simulink model "VCU_TDN"  (R2020a)
settings: Solver=FixedStepDiscrete  StartTime=0.0  StopTime=10.0  FixedStep=0.001  RelTol=1e-3  EnableMultiTasking=on
InitFcn:
  | EcoCoder_PreCheckLic();
undefined symbols (not defined in the file or in its folder): h, km
libraries: CoderSF_BSW_Libs x139, simulink x1, SF_CanService_Libs x1
(part 1 of 2)
settings Model: Creator=timot  LastModifiedBy=timot
settings DataIOCC: SaveFormat=Structure  SignalLoggingSaveFormat=ModelDataLogs  SaveOutput=off  SignalLogging=off  DSMLogging=off  SaveTime=off  ReturnWorkspaceOutputs=off
settings OptimizationCC: DefaultParameterBehavior=Inlined  InlineInvariantSignals=on  EnhancedBackFolding=on  StrengthReduction=on  EnableMemcpy=off  PassReuseOutputArgsAs=Individual arguments  EfficientFloat2IntCast=on  LifeSpan=1  SimCompilerOptimization=on  OptimizeBlockOrder=speed  DifferentSizesBufferReuse=on  EfficientTunableParamExpr=on
settings DebuggingCC: AlgebraicLoopMsg=none  ArtificialAlgebraicLoopMsg=none  SaveWithDisabledLinksMsg=none  SaveWithParameterizedLinksMsg=none  CheckSSInitialOutputMsg=off  UnderspecifiedInitializationDetection=Classic  SignalResolutionControl=TryResolveAll  BlockPriorityViolationMsg=error  MinStepSizeMsg=none  InheritedTsInSrcMsg=none  MultiTaskDSMMsg=none  MultiTaskCondExecSysMsg=none  MultiTaskRateTransMsg=warning  TasksWithSamePriorityMsg=none  SigSpecEnsureSampleTimeMsg=none  IntegerOverflowMsg=error  Int32ToFloatConvMsg=none  ParameterPrecisionLossMsg=none  ParameterTunabilityLossMsg=none  FixptConstOverflowMsg=error  FcnCallInpInsideContextMsg=warning  UnconnectedInputMsg=error  UnconnectedOutputMsg=error  UnconnectedLineMsg=error  FrameProcessingCompatibilityMsg=none  BusObjectLabelMismatch=none  RootOutportRequireBusObject=none  UnknownTsInhSupMsg=none  ModelReferenceDataLoggingMessage=none  OperatingPointInterfaceChecksumMismatchMsg=none  SFUnusedDataAndEventsDiag=none  SFUnexpectedBacktrackingDiag=none  SFInvalidInputDataAccessInChartInitDiag=none  SFNoUnconditionalDefaultTransitionDiag=none  SFTransitionOutsideNaturalParentDiag=none  SFUnreachableExecutionPathDiag=none  SFMachineParentedDataDiag=error
settings HardwareCC: ProdBitPerPointer=32  ProdBitPerSizeT=32  ProdBitPerPtrDiffT=32  ProdLargestAtomicInteger=Long  ProdLargestAtomicFloat=Double  ProdEndianess=BigEndian  ProdWordSize=32  ProdHWDeviceType=Freescale->MPC55xx
settings ModelReferenceCC: UpdateModelReferenceTargets=Force  ModelReferenceNumInstancesAllowed=Single  PropagateSignalLabelsOutOfModel=off
settings SFSimCC: SFSimEcho=off  MATLABDynamicMemAlloc=off
settings RTWCC: Description=Ecotrons MPC5xxx  SystemTargetFile=MPC5644A.tlc  GenerateMakefile=off  TemplateMakefile=ert_default_tmf  RTWVerbose=off  RetainRTWFile=on  RTWCompilerOptimization=on
settings CodeAppCC: IgnoreCustomStorageClasses=off  OperatorAnnotations=on  CustomSymbolStrGlobalVar=$N$M  CustomSymbolStrType=$N$M  CustomSymbolStrFcn=$N$M  CustomSymbolStrFcnArg=$N$M  CustomSymbolStrBlkIO=$N$M  CustomSymbolStrMacro=$N$M
settings STFCustomTargetCC: UtilityFuncGeneration=Shared location  MultiwordLength=256  IncludeMdlTerminateFcn=off  CombineOutputUpdateFcns=on  SuppressErrorStatus=on  ERTCustomFileBanners=on  SupportNonFinite=off  SupportComplex=off  SupportContinuousTime=off  SupportNonInlinedSFcns=off  MATLABClassNameForMDSCustomization=Simulink.SoftwareTarget.ERTCustomization  SystemTargetFile=MPC5644A.tlc
settings ERTTargetCC: UtilityFuncGeneration=Shared location  ParMdlRefBuildCompliant=off  CompOptLevelCompliant=off  ConcurrentExecutionCompliant=off  IncludeMdlTerminateFcn=off  SuppressErrorStatus=on  SupportNonFinite=off  SupportComplex=off  RemoveResetFunc=off  ModelStepFunctionPrototypeControlCompliant=off  CPPClassGenCompliant=off  UseToolchainInfoCompliant=off  GenerateASAP2=on  InlinedParameterPlacement=NonHierarchical  ERTCustomFileTemplate=MPC5644A_file_process.tlc  ERTFilePackagingFormat=Compact  PreserveIfCondition=on  ConvertIfToSwitch=off  PreserveExternInFcnDecls=off  SuppressUnreachableDefaultCases=off

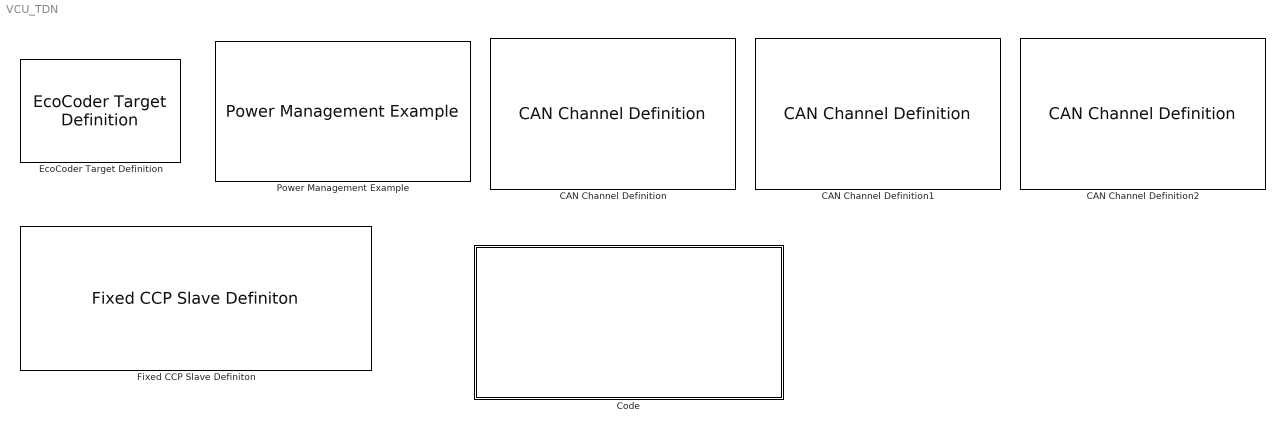
== system VCU_TDN ==
  CAN Channel Definition : CoderSF_BSW_Libs/CAN/CAN Channel Definition  Priority=2  channel=CAN_A  can_en=on  can_idfilter=off  can_rxextended=off  can_rxMask=hex2dec('7ff')  can_rxID=hex2dec('100')  can_baudrateIndex=500  can_txbuffer_size=20  can_rxbuffer_size=1  can_en_fd=off  nominalSamplePoint=7500  can_baudrateIndex_data=500  fastSamplePoint=7500  canfd_txbuffer_size=5  EcoCoderBlockID=C001_CANDef
  CAN Channel Definition1 : CoderSF_BSW_Libs/CAN/CAN Channel Definition  Priority=3  channel=CAN_B  can_en=on  can_idfilter=off  can_rxextended=off  can_rxMask=hex2dec('7ff')  can_rxID=hex2dec('100')  can_baudrateIndex=500  can_txbuffer_size=20  can_rxbuffer_size=1  can_en_fd=off  nominalSamplePoint=7500  can_baudrateIndex_data=500  fastSamplePoint=7500  canfd_txbuffer_size=5  EcoCoderBlockID=C001_CANDef
  CAN Channel Definition2 : CoderSF_BSW_Libs/CAN/CAN Channel Definition  Priority=4  channel=CAN_C  can_en=on  can_idfilter=off  can_rxextended=off  can_rxMask=hex2dec('7ff')  can_rxID=hex2dec('100')  can_baudrateIndex=500  can_txbuffer_size=20  can_rxbuffer_size=1  can_en_fd=off  nominalSamplePoint=7500  can_baudrateIndex_data=500  fastSamplePoint=7500  canfd_txbuffer_size=5  EcoCoderBlockID=C001_CANDef
  Code : Subsystem  Priority=6
  EcoCoder Target Definition : CoderSF_BSW_Libs/EcoCoder Target Definition  targetECU=EV2274A  EcoCoderBlockID=T001_Target  enNoTriggerCall=on  flgBlockReduction=on  flgShowDebugDisp=off  flgDisTargetOutFIleCounter=off  flgClearAllOldFiles=on  tc275_cal_len=hex2dec('00008000')  internal_flash=[hex2dec('00020000'),hex2dec('000E0000')]  cal_rom_phy=[hex2dec('00010000'),hex2dec('00002000')]  cal_ram_wp=[hex2dec('4000F000'),hex2dec('00002000')]  cal_ram_msm=[hex2dec('40000000'),hex2dec('00002000')]  var_ram_wp=[hex2dec('40002000'),hex2dec('0000D000')]  write_back_fixed_ram=[hex2dec('40011000'),hex2dec('00001000')]  write_back_unfixed_ram=[hex2dec('40012000'),hex2dec('00001000')]  stack=[hex2dec('40013000'),hex2dec('00001000')]
      settings: AttributesFormatString=Target :%<targetECU>
  Fixed CCP Slave Definiton : CoderSF_BSW_Libs/CCP/Fixed CCP Slave Definiton  Priority=5  ccpType=Configurable  ccp_enSet=on  ccp_disASW=on  channel=CAN_B  stationaddressSet=hex2dec('0112')  croidSet=hex2dec('100')  dtoidSet=hex2dec('101')  daqidSet=[hex2dec('101') hex2dec('101') hex2dec('101') hex2dec('102')]  daqpidSet=[hex2dec('0') hex2dec('3C') hex2dec('78') hex2dec('0')]  daqlenSet=[hex2dec('0') hex2dec('20') hex2dec('30') hex2dec('30')]  daqperSet=[5 20 100 0]  EcoCoderBlockID=C002_CCP21Conf
  Power Management Example : CoderSF_BSW_Libs/System Management Blocks/Power Management Example  Priority=1  flgKeyFromIn=off  tKeyOffDelaySet=0.5  flgResetSWEnSet=1  tDbncKeyOffFallSet=0.1  tDbncKeyOffRiseSet=1  facAd2VoltSet=109/27846  uKeyOffThrSet=1  uKeyOnHystSet=1  flgCANRxLiveCheckEn=0  flgEnPwrDwnFailReset=0  flgNVMEn=on  tShtDwnWait=500  flgPwrDwnByEdgeTrigger=off  EcoCoderBlockID=PME001_Def
      settings: AttributesFormatString=Priority:%<Priority>

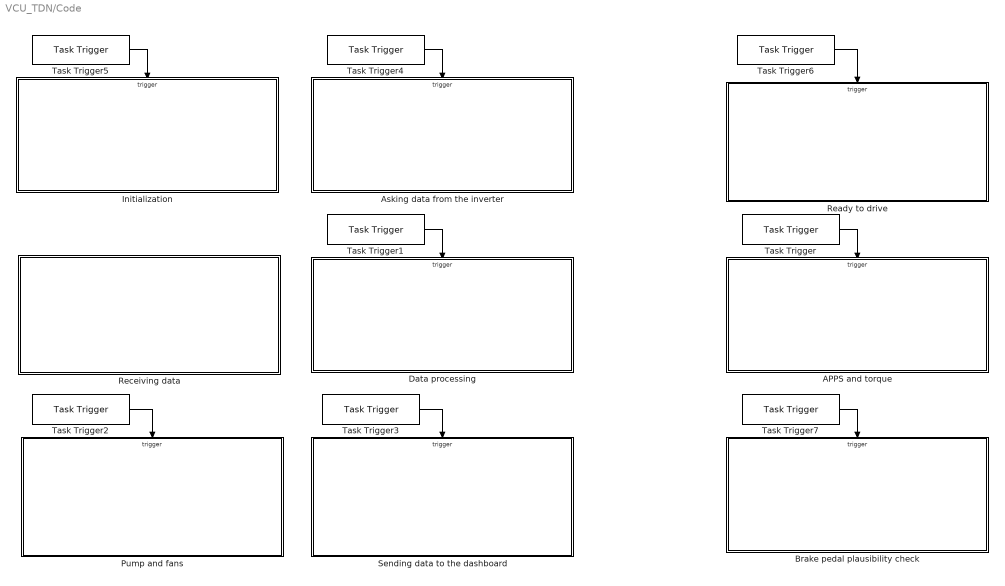
== system VCU_TDN/Code ==
  APPS and torque : Subsystem
  Asking data from the inverter : Subsystem
  Brake pedal plausibility check : Subsystem
  Data processing : Subsystem
  Initialization : Subsystem
  Pump and fans : Subsystem
  Ready to drive : Subsystem
  Receiving data : Subsystem
  Sending data to the dashboard : Subsystem
  Task Trigger : CoderSF_BSW_Libs/Task Scheduler/Task Trigger  tasktimeIndex=Task_H1ms
  Task Trigger1 : CoderSF_BSW_Libs/Task Scheduler/Task Trigger  tasktimeIndex=Task_L100ms
  Task Trigger2 : CoderSF_BSW_Libs/Task Scheduler/Task Trigger  tasktimeIndex=Task_L1000ms
  Task Trigger3 : CoderSF_BSW_Libs/Task Scheduler/Task Trigger  tasktimeIndex=Task_L100ms
  Task Trigger4 : CoderSF_BSW_Libs/Task Scheduler/Task Trigger  tasktimeIndex=Task_ini
  Task Trigger5 : CoderSF_BSW_Libs/Task Scheduler/Task Trigger  tasktimeIndex=Task_ini
  Task Trigger6 : CoderSF_BSW_Libs/Task Scheduler/Task Trigger  tasktimeIndex=Task_H1ms
  Task Trigger7 : CoderSF_BSW_Libs/Task Scheduler/Task Trigger  tasktimeIndex=Task_H1ms
  wires:
  Task Trigger/1 -> APPS and torque/Trigger
  Task Trigger3/1 -> Sending data to the dashboard/Trigger
  Task Trigger4/1 -> Asking data from the inverter/Trigger
  Task Trigger1/1 -> Data processing/Trigger
  Task Trigger2/1 -> Pump and fans/Trigger
  Task Trigger5/1 -> Initialization/Trigger
  Task Trigger6/1 -> Ready to drive/Trigger
  Task Trigger7/1 -> Brake pedal plausibility check/Trigger

== system VCU_TDN/Code/APPS and torque ==
  Trigger : TriggerPort  TriggerType=function-call  VariantControl=Variant  PortDimensions=1
  APPS 1 : CoderSF_BSW_Libs/ADC/Read ADC Value  channel=6
  APPS 2 : CoderSF_BSW_Libs/ADC/Read ADC Value  channel=7
  APPS Fault detection : Subsystem
  Throttle setpoint for the inverter : Subsystem
  wires:
  APPS 1/1 -> Throttle setpoint for the inverter/1(APPS 1), APPS Fault detection/1(APPS 1)
  APPS 2/1 -> Throttle setpoint for the inverter/2(APPS 2), APPS Fault detection/2(APPS 2)

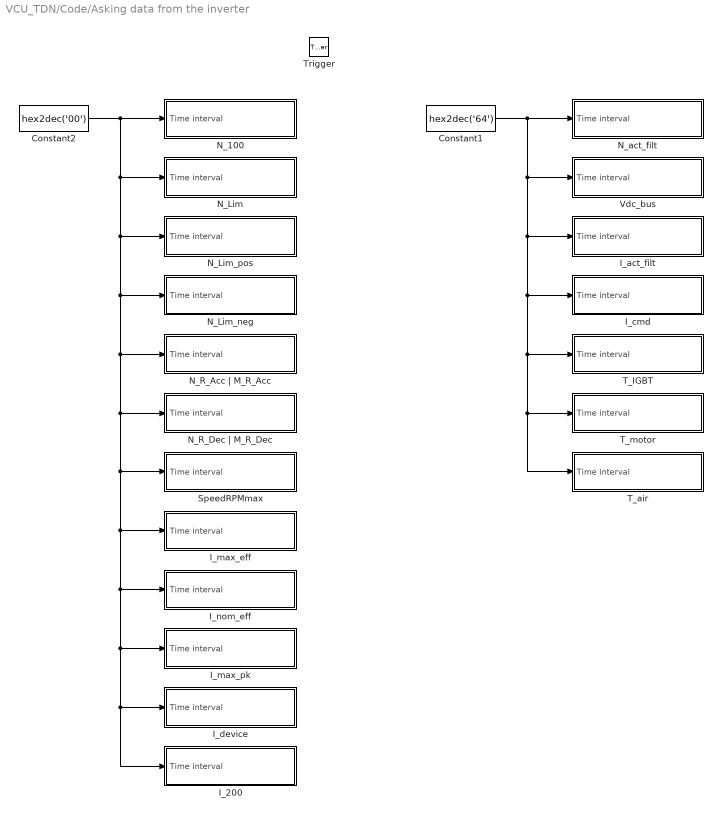
== system VCU_TDN/Code/Asking data from the inverter ==
  Trigger : TriggerPort  TriggerType=function-call  VariantControl=Variant  PortDimensions=1
  Constant1 : Constant  Value=hex2dec('64')  OutDataTypeStr=uint8
  Constant2 : Constant  Value=hex2dec('00')  OutDataTypeStr=uint8
  I_200 : Subsystem
  I_act_filt : Subsystem
  I_cmd : Subsystem
  I_device : Subsystem
  I_max_eff : Subsystem
  I_max_pk : Subsystem
  I_nom_eff : Subsystem
  N_100 : Subsystem
  N_Lim : Subsystem
  N_Lim_neg : Subsystem
  N_Lim_pos : Subsystem
  N_R_Acc | M_R_Acc : Subsystem
  N_R_Dec | M_R_Dec : Subsystem
  N_act_filt : Subsystem
  SpeedRPMmax : Subsystem
  T_IGBT : Subsystem
  T_air : Subsystem
  T_motor : Subsystem
  Vdc_bus : Subsystem
  wires:
  Constant2/1 -> SpeedRPMmax/1(Time interval), I_200/1(Time interval), I_device/1(Time interval), I_max_pk/1(Time interval), I_nom_eff/1(Time interval), I_max_eff/1(Time interval), N_R_Dec | M_R_Dec/1(Time interval), N_R_Acc | M_R_Acc/1(Time interval), N_Lim_neg/1(Time interval), N_Lim_pos/1(Time interval), N_Lim/1(Time interval), N_100/1(Time interval)
  Constant1/1 -> T_air/1(Time interval), T_motor/1(Time interval), T_IGBT/1(Time interval), I_cmd/1(Time interval), I_act_filt/1(Time interval), Vdc_bus/1(Time interval), N_act_filt/1(Time interval)

== system VCU_TDN/Code/Brake pedal plausibility check ==
  Trigger : TriggerPort  TriggerType=function-call  VariantControl=Variant  PortDimensions=1
  Logical Operator : Logic  AllPortsSameDT=off  OutDataTypeStr=boolean
  Read Calibration : CoderSF_BSW_Libs/Calibration & Measurement/Read Calibration  variable_name=BRAKE_CONTACTOR  variable_value=0  variable_type=boolean  variable_min=[]  variable_max=[]  unitStr=""  descStr=""
      settings: AttributesFormatString=value:%<variable_value> type:%<variable_type> max:%<variable_max> Min:%<variable_min>
  Read Calibration1 : CoderSF_BSW_Libs/Calibration & Measurement/Read Calibration  variable_name=APPS_M  variable_value=0  variable_type=boolean  variable_min=[]  variable_max=[]  unitStr=""  descStr=""
      settings: AttributesFormatString=value:%<variable_value> type:%<variable_type> max:%<variable_max> Min:%<variable_min>
  wires:
  Read Calibration1/1 -> Logical Operator/1
  Read Calibration/1 -> Logical Operator/2

== system VCU_TDN/Code/Data processing ==
  Trigger : TriggerPort  TriggerType=function-call  VariantControl=Variant  PortDimensions=1
  Current in the motor : Subsystem
  Speed : Subsystem

== system VCU_TDN/Code/Initialization ==
  Trigger : TriggerPort  TriggerType=function-call  VariantControl=Variant  PortDimensions=1
  Constant : Constant  Value=0  OutDataTypeStr=boolean
  Constant1 : Constant  Value=0  OutDataTypeStr=boolean
  Disabling the inverter : Subsystem
  FRG/RUN : CoderSF_BSW_Libs/Digital I//O/Switch Output  channel=LSO07
  RFE : CoderSF_BSW_Libs/Digital I//O/Switch Output  channel=LSO06
  wires:
  Constant/1 -> RFE/1
  Constant1/1 -> FRG/RUN/1

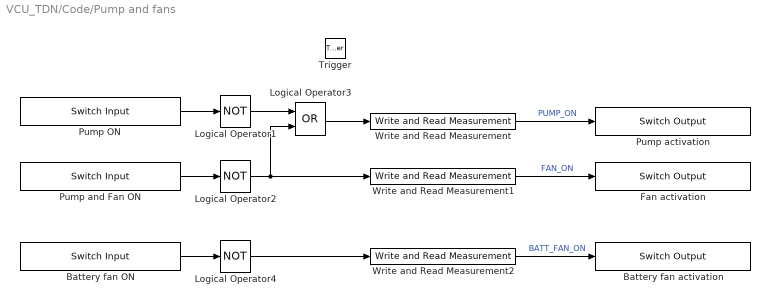
== system VCU_TDN/Code/Pump and fans ==
  Trigger : TriggerPort  TriggerType=function-call  VariantControl=Variant  PortDimensions=1
  Battery fan ON : CoderSF_BSW_Libs/Digital I//O/Switch Input  portNum=DI09
  Battery fan activation : CoderSF_BSW_Libs/Digital I//O/Switch Output  channel=LSO03
  Fan activation : CoderSF_BSW_Libs/Digital I//O/Switch Output  channel=LSO13
  Logical Operator1 : Logic  Operator=NOT  AllPortsSameDT=off  OutDataTypeStr=boolean
  Logical Operator2 : Logic  Operator=NOT  AllPortsSameDT=off  OutDataTypeStr=boolean
  Logical Operator3 : Logic  Operator=OR  AllPortsSameDT=off  OutDataTypeStr=boolean
  Logical Operator4 : Logic  Operator=NOT  AllPortsSameDT=off  OutDataTypeStr=boolean
  Pump ON : CoderSF_BSW_Libs/Digital I//O/Switch Input  portNum=DI12
  Pump activation : CoderSF_BSW_Libs/Digital I//O/Switch Output  channel=LSO12
  Pump and Fan ON : CoderSF_BSW_Libs/Digital I//O/Switch Input  portNum=DI12
  Write and Read Measurement : CoderSF_BSW_Libs/Calibration & Measurement/Write and Read Measurement  variable_name=PUMP_ON  variable_value=0  variable_type=boolean  numD=1  unitStr=""  descStr=""
      settings: AttributesFormatString=type:%<variable_type> Dimensions:%<numD>
  Write and Read Measurement1 : CoderSF_BSW_Libs/Calibration & Measurement/Write and Read Measurement  variable_name=FAN_ON  variable_value=0  variable_type=boolean  numD=1  unitStr=""  descStr=""
      settings: AttributesFormatString=type:%<variable_type> Dimensions:%<numD>
  Write and Read Measurement2 : CoderSF_BSW_Libs/Calibration & Measurement/Write and Read Measurement  variable_name=BATT_FAN_ON  variable_value=0  variable_type=boolean  numD=1  unitStr=""  descStr=""
      settings: AttributesFormatString=type:%<variable_type> Dimensions:%<numD>
  wires:
  Logical Operator2/1 -> Write and Read Measurement1/1, Logical Operator3/2
  Pump and Fan ON/1 -> Logical Operator2/1
  Logical Operator1/1 -> Logical Operator3/1
  Logical Operator4/1 -> Write and Read Measurement2/1
  Logical Operator3/1 -> Write and Read Measurement/1
  Battery fan ON/1 -> Logical Operator4/1
  Pump ON/1 -> Logical Operator1/1
  Write and Read Measurement2/1 -> Battery fan activation/1  "BATT_FAN_ON"
  Write and Read Measurement1/1 -> Fan activation/1  "FAN_ON"
  Write and Read Measurement/1 -> Pump activation/1  "PUMP_ON"

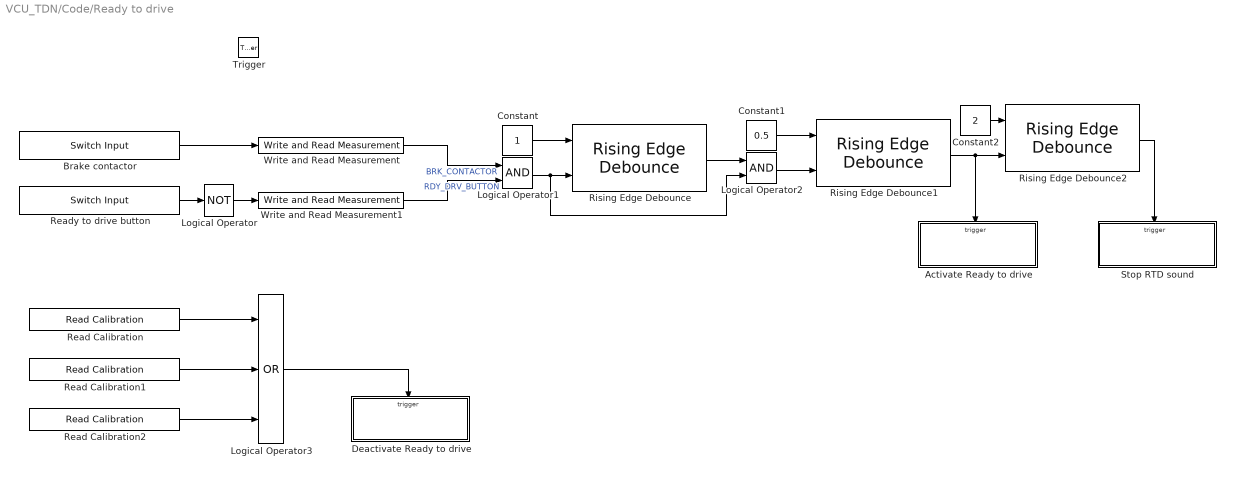
== system VCU_TDN/Code/Ready to drive ==
  Trigger : TriggerPort  TriggerType=function-call  VariantControl=Variant  PortDimensions=1
  Activate Ready to drive : Subsystem  TreatAsAtomicUnit=on
  Brake contactor : CoderSF_BSW_Libs/Digital I//O/Switch Input  portNum=DI18
  Constant : Constant  OutDataTypeStr=Inherit: Inherit via back propagation
  Constant1 : Constant  Value=0.5  OutDataTypeStr=Inherit: Inherit via back propagation
  Constant2 : Constant  Value=2  OutDataTypeStr=Inherit: Inherit via back propagation
  Deactivate Ready to drive : Subsystem  TreatAsAtomicUnit=on
  Logical Operator : Logic  Operator=NOT  AllPortsSameDT=off  OutDataTypeStr=boolean
  Logical Operator1 : Logic  AllPortsSameDT=off  OutDataTypeStr=boolean
  Logical Operator2 : Logic  AllPortsSameDT=off  OutDataTypeStr=boolean
  Logical Operator3 : Logic  Operator=OR  Inputs=3  AllPortsSameDT=off  OutDataTypeStr=boolean
  Read Calibration : CoderSF_BSW_Libs/Calibration & Measurement/Read Calibration  variable_name=APPS_FAULT  variable_value=0  variable_type=boolean  variable_min=[]  variable_max=[]  unitStr=""  descStr=""
      settings: AttributesFormatString=value:%<variable_value> type:%<variable_type> max:%<variable_max> Min:%<variable_min>
  Read Calibration1 : CoderSF_BSW_Libs/Calibration & Measurement/Read Calibration  variable_name=BRK_PDL_FAULT  variable_value=0  variable_type=boolean  variable_min=[]  variable_max=[]  unitStr=""  descStr=""
      settings: AttributesFormatString=value:%<variable_value> type:%<variable_type> max:%<variable_max> Min:%<variable_min>
  Read Calibration2 : CoderSF_BSW_Libs/Calibration & Measurement/Read Calibration  variable_name=INV_DIS  variable_value=0  variable_type=boolean  variable_min=[]  variable_max=[]  unitStr=""  descStr=""
      settings: AttributesFormatString=value:%<variable_value> type:%<variable_type> max:%<variable_max> Min:%<variable_min>
  Ready to drive button : CoderSF_BSW_Libs/Digital I//O/Switch Input  portNum=DI01
  Rising Edge Debounce : CoderSF_BSW_Libs/Application Base Blocks/Rising Edge Debounce  ic=off
  Rising Edge Debounce1 : CoderSF_BSW_Libs/Application Base Blocks/Rising Edge Debounce  ic=off
  Rising Edge Debounce2 : CoderSF_BSW_Libs/Application Base Blocks/Rising Edge Debounce  ic=off
  Stop RTD sound : Subsystem  TreatAsAtomicUnit=on
  Write and Read Measurement : CoderSF_BSW_Libs/Calibration & Measurement/Write and Read Measurement  variable_name=BRK_CONTACTOR  variable_value=0  variable_type=boolean  numD=1  unitStr=""  descStr=""
      settings: AttributesFormatString=type:%<variable_type> Dimensions:%<numD>
  Write and Read Measurement1 : CoderSF_BSW_Libs/Calibration & Measurement/Write and Read Measurement  variable_name=RDY_DRV_BUTTON  variable_value=0  variable_type=boolean  numD=1  unitStr=""  descStr=""
      settings: AttributesFormatString=type:%<variable_type> Dimensions:%<numD>
  wires:
  Ready to drive button/1 -> Logical Operator/1
  Brake contactor/1 -> Write and Read Measurement/1
  Logical Operator/1 -> Write and Read Measurement1/1
  Write and Read Measurement/1 -> Logical Operator1/1  "BRK_CONTACTOR"
  Write and Read Measurement1/1 -> Logical Operator1/2  "RDY_DRV_BUTTON"
  Logical Operator1/1 -> Logical Operator2/2, Rising Edge Debounce/2
  Constant/1 -> Rising Edge Debounce/1
  Rising Edge Debounce/1 -> Logical Operator2/1
  Read Calibration/1 -> Logical Operator3/1
  Logical Operator3/1 -> Deactivate Ready to drive/Trigger
  Read Calibration1/1 -> Logical Operator3/2
  Read Calibration2/1 -> Logical Operator3/3
  Constant1/1 -> Rising Edge Debounce1/1
  Rising Edge Debounce1/1 -> Rising Edge Debounce2/2, Activate Ready to drive/Trigger
  Logical Operator2/1 -> Rising Edge Debounce1/2
  Constant2/1 -> Rising Edge Debounce2/1
  Rising Edge Debounce2/1 -> Stop RTD sound/Trigger

== system VCU_TDN/Code/Receiving data ==
  BMS : Subsystem
  Battery temperature sensors : Subsystem
  Inverter : Subsystem
  Sensors : Subsystem
  Task Trigger1 : CoderSF_BSW_Libs/Task Scheduler/Task Trigger  tasktimeIndex=Task_L100ms
  wires:
  Task Trigger1/1 -> Sensors/Trigger

== system VCU_TDN/Code/Sending data to the dashboard ==
  Trigger : TriggerPort  TriggerType=function-call  VariantControl=Variant  PortDimensions=1
  Read Calibration : CoderSF_BSW_Libs/Calibration & Measurement/Read Calibration  variable_name=Speed  variable_value=0  variable_type=int16  variable_min=[]  variable_max=[]  unitStr=km/h  descStr=""
      settings: AttributesFormatString=value:%<variable_value> type:%<variable_type> max:%<variable_max> Min:%<variable_min>
  Read Calibration1 : CoderSF_BSW_Libs/Calibration & Measurement/Read Calibration  variable_name=Temp_batt_HV  variable_value=0  variable_type=uint8  variable_min=[]  variable_max=[]  unitStr=°C  descStr=""
      settings: AttributesFormatString=value:%<variable_value> type:%<variable_type> max:%<variable_max> Min:%<variable_min>
  Read Calibration2 : CoderSF_BSW_Libs/Calibration & Measurement/Read Calibration  variable_name=SOC_batt_HV  variable_value=0  variable_type=uint8  variable_min=[]  variable_max=[]  descStr=""
      settings: AttributesFormatString=value:%<variable_value> type:%<variable_type> max:%<variable_max> Min:%<variable_min>
  Terminator : Terminator
  Terminator1 : Terminator
  Terminator2 : Terminator
  wires:
  Read Calibration/1 -> Terminator/1
  Read Calibration1/1 -> Terminator1/1
  Read Calibration2/1 -> Terminator2/1

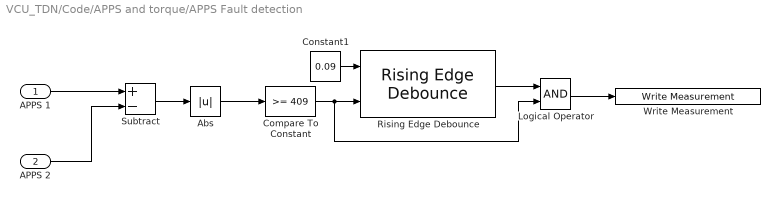
== system VCU_TDN/Code/APPS and torque/APPS Fault detection ==
  APPS 1 : Inport
  APPS 2 : Inport  Port=2
  Abs : Abs
  Compare To Constant : simulink/Logic and Bit Operations/Compare To Constant  relop=>=  const=409  OutDataTypeStr=boolean
  Constant1 : Constant  Value=0.09  OutDataTypeStr=Inherit: Inherit via back propagation
  Logical Operator : Logic  AllPortsSameDT=off  OutDataTypeStr=boolean
  Rising Edge Debounce : CoderSF_BSW_Libs/Application Base Blocks/Rising Edge Debounce  ic=off
  Subtract : Sum  Inputs=+-
  Write Measurement : CoderSF_BSW_Libs/Calibration & Measurement/Write Measurement  variable_name=APPS_FAULT  variable_value=0  variable_type=boolean  numD=1  unitStr=""  descStr=""
      settings: AttributesFormatString=type:%<variable_type> Dimensions:%<numD>
  wires:
  APPS 1/1 -> Subtract/1
  Subtract/1 -> Abs/1
  Constant1/1 -> Rising Edge Debounce/1
  Compare To Constant/1 -> Logical Operator/2, Rising Edge Debounce/2
  Abs/1 -> Compare To Constant/1
  Logical Operator/1 -> Write Measurement/1
  APPS 2/1 -> Subtract/2
  Rising Edge Debounce/1 -> Logical Operator/1

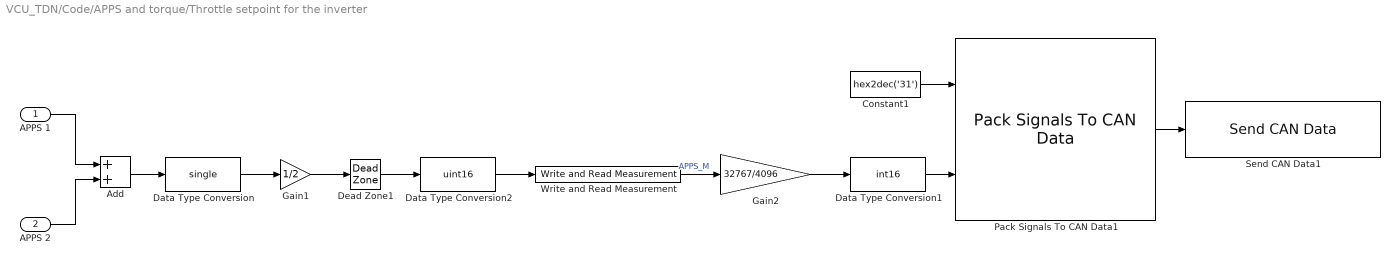
== system VCU_TDN/Code/APPS and torque/Throttle setpoint for the inverter ==
  APPS 1 : Inport
  APPS 2 : Inport  Port=2
  Add : Sum
  Constant1 : Constant  Value=hex2dec('31')  OutDataTypeStr=uint8
  Data Type Conversion : DataTypeConversion  OutDataTypeStr=single
  Data Type Conversion1 : DataTypeConversion  OutDataTypeStr=int16
  Data Type Conversion2 : DataTypeConversion  OutDataTypeStr=uint16
  Dead Zone1 : DeadZone  LowerValue=-5  UpperValue=5  SaturateOnIntegerOverflow=on
  Gain1 : Gain  Gain=1/2
  Gain2 : Gain  Gain=32767/4096
  Pack Signals To CAN Data1 : CoderSF_BSW_Libs/CAN/Pack Signals To CAN Data  Signal="{{'REG_31'  'Data1'},[0 8],[8 16],{'uint8'  'int16'},{'Intel' 'Intel'}}"
  Send CAN Data1 : CoderSF_BSW_Libs/CAN/Send CAN Data  channel=CAN_A  txlen=3  txid=hex2dec('201')  frametype=Standard(11-bit ID)  showerror=off
  Write and Read Measurement : CoderSF_BSW_Libs/Calibration & Measurement/Write and Read Measurement  variable_name=APPS_M  variable_value=0  variable_type=uint16  numD=1  unitStr=""  descStr=""
      settings: AttributesFormatString=type:%<variable_type> Dimensions:%<numD>
  wires:
  APPS 1/1 -> Add/1
  Gain1/1 -> Dead Zone1/1
  Pack Signals To CAN Data1/1 -> Send CAN Data1/1
  Add/1 -> Data Type Conversion/1
  Gain2/1 -> Data Type Conversion1/1
  Data Type Conversion1/1 -> Pack Signals To CAN Data1/2
  Constant1/1 -> Pack Signals To CAN Data1/1
  Data Type Conversion/1 -> Gain1/1
  APPS 2/1 -> Add/2
  Write and Read Measurement/1 -> Gain2/1  "APPS_M"
  Dead Zone1/1 -> Data Type Conversion2/1
  Data Type Conversion2/1 -> Write and Read Measurement/1

== system VCU_TDN/Code/Asking data from the inverter/I_200 ==
  Time interval : Inport
  Constant : Constant  Value=hex2dec('3d')  OutDataTypeStr=uint8
  Constant1 : Constant  Value=hex2dec('d9')  OutDataTypeStr=uint8
  Pack Signals To CAN Data : CoderSF_BSW_Libs/CAN/Pack Signals To CAN Data  Signal="{{'REG_31'  'Data1' 'Data2'},[0 8 16],[8 8 8],{'uint8'  'uint8' 'uint8'},{'Intel' 'Intel' 'Intel'}}"
  Send CAN Data : CoderSF_BSW_Libs/CAN/Send CAN Data  channel=CAN_A  txlen=3  txid=hex2dec('201')  frametype=Standard(11-bit ID)  showerror=off
  wires:
  Constant/1 -> Pack Signals To CAN Data/1
  Pack Signals To CAN Data/1 -> Send CAN Data/1
  Constant1/1 -> Pack Signals To CAN Data/2
  Time interval/1 -> Pack Signals To CAN Data/3

== system VCU_TDN/Code/Asking data from the inverter/I_act_filt ==
  Time interval : Inport
  Constant : Constant  Value=hex2dec('3d')  OutDataTypeStr=uint8
  Constant1 : Constant  Value=hex2dec('5f')  OutDataTypeStr=uint8
  Pack Signals To CAN Data : CoderSF_BSW_Libs/CAN/Pack Signals To CAN Data  Signal="{{'REG_31'  'Data1' 'Data2'},[0 8 16],[8 8 8],{'uint8'  'uint8' 'uint8'},{'Intel' 'Intel' 'Intel'}}"
  Send CAN Data : CoderSF_BSW_Libs/CAN/Send CAN Data  channel=CAN_A  txlen=3  txid=hex2dec('201')  frametype=Standard(11-bit ID)  showerror=off
  wires:
  Constant/1 -> Pack Signals To CAN Data/1
  Pack Signals To CAN Data/1 -> Send CAN Data/1
  Constant1/1 -> Pack Signals To CAN Data/2
  Time interval/1 -> Pack Signals To CAN Data/3

== system VCU_TDN/Code/Asking data from the inverter/I_cmd ==
  Time interval : Inport
  Constant : Constant  Value=hex2dec('3d')  OutDataTypeStr=uint8
  Constant1 : Constant  Value=hex2dec('26')  OutDataTypeStr=uint8
  Pack Signals To CAN Data : CoderSF_BSW_Libs/CAN/Pack Signals To CAN Data  Signal="{{'REG_31'  'Data1' 'Data2'},[0 8 16],[8 8 8],{'uint8'  'uint8' 'uint8'},{'Intel' 'Intel' 'Intel'}}"
  Send CAN Data : CoderSF_BSW_Libs/CAN/Send CAN Data  channel=CAN_A  txlen=3  txid=hex2dec('201')  frametype=Standard(11-bit ID)  showerror=off
  wires:
  Constant/1 -> Pack Signals To CAN Data/1
  Pack Signals To CAN Data/1 -> Send CAN Data/1
  Constant1/1 -> Pack Signals To CAN Data/2
  Time interval/1 -> Pack Signals To CAN Data/3

== system VCU_TDN/Code/Asking data from the inverter/I_device ==
  Time interval : Inport
  Constant : Constant  Value=hex2dec('3d')  OutDataTypeStr=uint8
  Constant1 : Constant  Value=hex2dec('c6')  OutDataTypeStr=uint8
  Pack Signals To CAN Data : CoderSF_BSW_Libs/CAN/Pack Signals To CAN Data  Signal="{{'REG_31'  'Data1' 'Data2'},[0 8 16],[8 8 8],{'uint8'  'uint8' 'uint8'},{'Intel' 'Intel' 'Intel'}}"
  Send CAN Data : CoderSF_BSW_Libs/CAN/Send CAN Data  channel=CAN_A  txlen=3  txid=hex2dec('201')  frametype=Standard(11-bit ID)  showerror=off
  wires:
  Constant/1 -> Pack Signals To CAN Data/1
  Pack Signals To CAN Data/1 -> Send CAN Data/1
  Constant1/1 -> Pack Signals To CAN Data/2
  Time interval/1 -> Pack Signals To CAN Data/3

== system VCU_TDN/Code/Asking data from the inverter/I_max_eff ==
  Time interval : Inport
  Constant : Constant  Value=hex2dec('3d')  OutDataTypeStr=uint8
  Constant1 : Constant  Value=hex2dec('4d')  OutDataTypeStr=uint8
  Pack Signals To CAN Data : CoderSF_BSW_Libs/CAN/Pack Signals To CAN Data  Signal="{{'REG_31'  'Data1' 'Data2'},[0 8 16],[8 8 8],{'uint8'  'uint8' 'uint8'},{'Intel' 'Intel' 'Intel'}}"
  Send CAN Data : CoderSF_BSW_Libs/CAN/Send CAN Data  channel=CAN_A  txlen=3  txid=hex2dec('201')  frametype=Standard(11-bit ID)  showerror=off
  wires:
  Constant/1 -> Pack Signals To CAN Data/1
  Pack Signals To CAN Data/1 -> Send CAN Data/1
  Constant1/1 -> Pack Signals To CAN Data/2
  Time interval/1 -> Pack Signals To CAN Data/3

== system VCU_TDN/Code/Asking data from the inverter/I_max_pk ==
  Time interval : Inport
  Constant : Constant  Value=hex2dec('3d')  OutDataTypeStr=uint8
  Constant1 : Constant  Value=hex2dec('c4')  OutDataTypeStr=uint8
  Pack Signals To CAN Data : CoderSF_BSW_Libs/CAN/Pack Signals To CAN Data  Signal="{{'REG_31'  'Data1' 'Data2'},[0 8 16],[8 8 8],{'uint8'  'uint8' 'uint8'},{'Intel' 'Intel' 'Intel'}}"
  Send CAN Data : CoderSF_BSW_Libs/CAN/Send CAN Data  channel=CAN_A  txlen=3  txid=hex2dec('201')  frametype=Standard(11-bit ID)  showerror=off
  wires:
  Constant/1 -> Pack Signals To CAN Data/1
  Pack Signals To CAN Data/1 -> Send CAN Data/1
  Constant1/1 -> Pack Signals To CAN Data/2
  Time interval/1 -> Pack Signals To CAN Data/3

== system VCU_TDN/Code/Asking data from the inverter/I_nom_eff ==
  Time interval : Inport
  Constant : Constant  Value=hex2dec('3d')  OutDataTypeStr=uint8
  Constant1 : Constant  Value=hex2dec('4e')  OutDataTypeStr=uint8
  Pack Signals To CAN Data : CoderSF_BSW_Libs/CAN/Pack Signals To CAN Data  Signal="{{'REG_31'  'Data1' 'Data2'},[0 8 16],[8 8 8],{'uint8'  'uint8' 'uint8'},{'Intel' 'Intel' 'Intel'}}"
  Send CAN Data : CoderSF_BSW_Libs/CAN/Send CAN Data  channel=CAN_A  txlen=3  txid=hex2dec('201')  frametype=Standard(11-bit ID)  showerror=off
  wires:
  Constant/1 -> Pack Signals To CAN Data/1
  Pack Signals To CAN Data/1 -> Send CAN Data/1
  Constant1/1 -> Pack Signals To CAN Data/2
  Time interval/1 -> Pack Signals To CAN Data/3

== system VCU_TDN/Code/Asking data from the inverter/N_100 ==
  Time interval : Inport
  Constant : Constant  Value=hex2dec('3d')  OutDataTypeStr=uint8
  Constant1 : Constant  Value=hex2dec('c8')  OutDataTypeStr=uint8
  Pack Signals To CAN Data : CoderSF_BSW_Libs/CAN/Pack Signals To CAN Data  Signal="{{'REG_31'  'Data1' 'Data2'},[0 8 16],[8 8 8],{'uint8'  'uint8' 'uint8'},{'Intel' 'Intel' 'Intel'}}"
  Send CAN Data : CoderSF_BSW_Libs/CAN/Send CAN Data  channel=CAN_A  txlen=3  txid=hex2dec('201')  frametype=Standard(11-bit ID)  showerror=off
  wires:
  Constant/1 -> Pack Signals To CAN Data/1
  Pack Signals To CAN Data/1 -> Send CAN Data/1
  Constant1/1 -> Pack Signals To CAN Data/2
  Time interval/1 -> Pack Signals To CAN Data/3

== system VCU_TDN/Code/Asking data from the inverter/N_Lim ==
  Time interval : Inport
  Constant : Constant  Value=hex2dec('3d')  OutDataTypeStr=uint8
  Constant1 : Constant  Value=hex2dec('34')  OutDataTypeStr=uint8
  Pack Signals To CAN Data : CoderSF_BSW_Libs/CAN/Pack Signals To CAN Data  Signal="{{'REG_31'  'Data1' 'Data2'},[0 8 16],[8 8 8],{'uint8'  'uint8' 'uint8'},{'Intel' 'Intel' 'Intel'}}"
  Send CAN Data : CoderSF_BSW_Libs/CAN/Send CAN Data  channel=CAN_A  txlen=3  txid=hex2dec('201')  frametype=Standard(11-bit ID)  showerror=off
  wires:
  Constant/1 -> Pack Signals To CAN Data/1
  Pack Signals To CAN Data/1 -> Send CAN Data/1
  Constant1/1 -> Pack Signals To CAN Data/2
  Time interval/1 -> Pack Signals To CAN Data/3

== system VCU_TDN/Code/Asking data from the inverter/N_Lim_neg ==
  Time interval : Inport
  Constant : Constant  Value=hex2dec('3d')  OutDataTypeStr=uint8
  Constant1 : Constant  Value=hex2dec('3e')  OutDataTypeStr=uint8
  Pack Signals To CAN Data : CoderSF_BSW_Libs/CAN/Pack Signals To CAN Data  Signal="{{'REG_31'  'Data1' 'Data2'},[0 8 16],[8 8 8],{'uint8'  'uint8' 'uint8'},{'Intel' 'Intel' 'Intel'}}"
  Send CAN Data : CoderSF_BSW_Libs/CAN/Send CAN Data  channel=CAN_A  txlen=3  txid=hex2dec('201')  frametype=Standard(11-bit ID)  showerror=off
  wires:
  Constant/1 -> Pack Signals To CAN Data/1
  Pack Signals To CAN Data/1 -> Send CAN Data/1
  Constant1/1 -> Pack Signals To CAN Data/2
  Time interval/1 -> Pack Signals To CAN Data/3

== system VCU_TDN/Code/Asking data from the inverter/N_Lim_pos ==
  Time interval : Inport
  Constant : Constant  Value=hex2dec('3d')  OutDataTypeStr=uint8
  Constant1 : Constant  Value=hex2dec('3f')  OutDataTypeStr=uint8
  Pack Signals To CAN Data : CoderSF_BSW_Libs/CAN/Pack Signals To CAN Data  Signal="{{'REG_31'  'Data1' 'Data2'},[0 8 16],[8 8 8],{'uint8'  'uint8' 'uint8'},{'Intel' 'Intel' 'Intel'}}"
  Send CAN Data : CoderSF_BSW_Libs/CAN/Send CAN Data  channel=CAN_A  txlen=3  txid=hex2dec('201')  frametype=Standard(11-bit ID)  showerror=off
  wires:
  Constant/1 -> Pack Signals To CAN Data/1
  Pack Signals To CAN Data/1 -> Send CAN Data/1
  Constant1/1 -> Pack Signals To CAN Data/2
  Time interval/1 -> Pack Signals To CAN Data/3

== system VCU_TDN/Code/Asking data from the inverter/N_R_Acc | M_R_Acc ==
  Time interval : Inport
  Constant : Constant  Value=hex2dec('3d')  OutDataTypeStr=uint8
  Constant1 : Constant  Value=hex2dec('35')  OutDataTypeStr=uint8
  Pack Signals To CAN Data : CoderSF_BSW_Libs/CAN/Pack Signals To CAN Data  Signal="{{'REG_31'  'Data1' 'Data2'},[0 8 16],[8 8 8],{'uint8'  'uint8' 'uint8'},{'Intel' 'Intel' 'Intel'}}"
  Send CAN Data : CoderSF_BSW_Libs/CAN/Send CAN Data  channel=CAN_A  txlen=3  txid=hex2dec('201')  frametype=Standard(11-bit ID)  showerror=off
  wires:
  Constant/1 -> Pack Signals To CAN Data/1
  Pack Signals To CAN Data/1 -> Send CAN Data/1
  Constant1/1 -> Pack Signals To CAN Data/2
  Time interval/1 -> Pack Signals To CAN Data/3

== system VCU_TDN/Code/Asking data from the inverter/N_R_Dec | M_R_Dec ==
  Time interval : Inport
  Constant : Constant  Value=hex2dec('3d')  OutDataTypeStr=uint8
  Constant1 : Constant  Value=hex2dec('ed')  OutDataTypeStr=uint8
  Pack Signals To CAN Data : CoderSF_BSW_Libs/CAN/Pack Signals To CAN Data  Signal="{{'REG_31'  'Data1' 'Data2'},[0 8 16],[8 8 8],{'uint8'  'uint8' 'uint8'},{'Intel' 'Intel' 'Intel'}}"
  Send CAN Data : CoderSF_BSW_Libs/CAN/Send CAN Data  channel=CAN_A  txlen=3  txid=hex2dec('201')  frametype=Standard(11-bit ID)  showerror=off
  wires:
  Constant/1 -> Pack Signals To CAN Data/1
  Pack Signals To CAN Data/1 -> Send CAN Data/1
  Constant1/1 -> Pack Signals To CAN Data/2
  Time interval/1 -> Pack Signals To CAN Data/3

== system VCU_TDN/Code/Asking data from the inverter/N_act_filt ==
  Time interval : Inport
  Constant : Constant  Value=hex2dec('3d')  OutDataTypeStr=uint8
  Constant1 : Constant  Value=hex2dec('a8')  OutDataTypeStr=uint8
  Pack Signals To CAN Data : CoderSF_BSW_Libs/CAN/Pack Signals To CAN Data  Signal="{{'REG_31'  'Data1' 'Data2'},[0 8 16],[8 8 8],{'uint8'  'uint8' 'uint8'},{'Intel' 'Intel' 'Intel'}}"
  Send CAN Data : CoderSF_BSW_Libs/CAN/Send CAN Data  channel=CAN_A  txlen=3  txid=hex2dec('201')  frametype=Standard(11-bit ID)  showerror=off
  wires:
  Constant/1 -> Pack Signals To CAN Data/1
  Pack Signals To CAN Data/1 -> Send CAN Data/1
  Constant1/1 -> Pack Signals To CAN Data/2
  Time interval/1 -> Pack Signals To CAN Data/3

== system VCU_TDN/Code/Asking data from the inverter/SpeedRPMmax ==
  Time interval : Inport
  Constant : Constant  Value=hex2dec('3d')  OutDataTypeStr=uint8
  Constant1 : Constant  Value=hex2dec('ce')  OutDataTypeStr=uint8
  Pack Signals To CAN Data : CoderSF_BSW_Libs/CAN/Pack Signals To CAN Data  Signal="{{'REG_31'  'Data1' 'Data2'},[0 8 16],[8 8 8],{'uint8'  'uint8' 'uint8'},{'Intel' 'Intel' 'Intel'}}"
  Send CAN Data : CoderSF_BSW_Libs/CAN/Send CAN Data  channel=CAN_A  txlen=3  txid=hex2dec('201')  frametype=Standard(11-bit ID)  showerror=off
  wires:
  Constant/1 -> Pack Signals To CAN Data/1
  Pack Signals To CAN Data/1 -> Send CAN Data/1
  Constant1/1 -> Pack Signals To CAN Data/2
  Time interval/1 -> Pack Signals To CAN Data/3

== system VCU_TDN/Code/Asking data from the inverter/T_IGBT ==
  Time interval : Inport
  Constant : Constant  Value=hex2dec('3d')  OutDataTypeStr=uint8
  Constant1 : Constant  Value=hex2dec('4a')  OutDataTypeStr=uint8
  Pack Signals To CAN Data : CoderSF_BSW_Libs/CAN/Pack Signals To CAN Data  Signal="{{'REG_31'  'Data1' 'Data2'},[0 8 16],[8 8 8],{'uint8'  'uint8' 'uint8'},{'Intel' 'Intel' 'Intel'}}"
  Send CAN Data : CoderSF_BSW_Libs/CAN/Send CAN Data  channel=CAN_A  txlen=3  txid=hex2dec('201')  frametype=Standard(11-bit ID)  showerror=off
  wires:
  Constant/1 -> Pack Signals To CAN Data/1
  Pack Signals To CAN Data/1 -> Send CAN Data/1
  Constant1/1 -> Pack Signals To CAN Data/2
  Time interval/1 -> Pack Signals To CAN Data/3

== system VCU_TDN/Code/Asking data from the inverter/T_air ==
  Time interval : Inport
  Constant : Constant  Value=hex2dec('3d')  OutDataTypeStr=uint8
  Constant1 : Constant  Value=hex2dec('4b')  OutDataTypeStr=uint8
  Pack Signals To CAN Data : CoderSF_BSW_Libs/CAN/Pack Signals To CAN Data  Signal="{{'REG_31'  'Data1' 'Data2'},[0 8 16],[8 8 8],{'uint8'  'uint8' 'uint8'},{'Intel' 'Intel' 'Intel'}}"
  Send CAN Data : CoderSF_BSW_Libs/CAN/Send CAN Data  channel=CAN_A  txlen=3  txid=hex2dec('201')  frametype=Standard(11-bit ID)  showerror=off
  wires:
  Constant/1 -> Pack Signals To CAN Data/1
  Pack Signals To CAN Data/1 -> Send CAN Data/1
  Constant1/1 -> Pack Signals To CAN Data/2
  Time interval/1 -> Pack Signals To CAN Data/3

== system VCU_TDN/Code/Asking data from the inverter/T_motor ==
  Time interval : Inport
  Constant : Constant  Value=hex2dec('3d')  OutDataTypeStr=uint8
  Constant1 : Constant  Value=hex2dec('49')  OutDataTypeStr=uint8
  Pack Signals To CAN Data : CoderSF_BSW_Libs/CAN/Pack Signals To CAN Data  Signal="{{'REG_31'  'Data1' 'Data2'},[0 8 16],[8 8 8],{'uint8'  'uint8' 'uint8'},{'Intel' 'Intel' 'Intel'}}"
  Send CAN Data : CoderSF_BSW_Libs/CAN/Send CAN Data  channel=CAN_A  txlen=3  txid=hex2dec('201')  frametype=Standard(11-bit ID)  showerror=off
  wires:
  Constant/1 -> Pack Signals To CAN Data/1
  Pack Signals To CAN Data/1 -> Send CAN Data/1
  Constant1/1 -> Pack Signals To CAN Data/2
  Time interval/1 -> Pack Signals To CAN Data/3

== system VCU_TDN/Code/Asking data from the inverter/Vdc_bus ==
  Time interval : Inport
  Constant : Constant  Value=hex2dec('3d')  OutDataTypeStr=uint8
  Constant1 : Constant  Value=hex2dec('eb')  OutDataTypeStr=uint8
  Pack Signals To CAN Data : CoderSF_BSW_Libs/CAN/Pack Signals To CAN Data  Signal="{{'REG_31'  'Data1' 'Data2'},[0 8 16],[8 8 8],{'uint8'  'uint8' 'uint8'},{'Intel' 'Intel' 'Intel'}}"
  Send CAN Data : CoderSF_BSW_Libs/CAN/Send CAN Data  channel=CAN_A  txlen=3  txid=hex2dec('201')  frametype=Standard(11-bit ID)  showerror=off
  wires:
  Constant/1 -> Pack Signals To CAN Data/1
  Pack Signals To CAN Data/1 -> Send CAN Data/1
  Constant1/1 -> Pack Signals To CAN Data/2
  Time interval/1 -> Pack Signals To CAN Data/3

== system VCU_TDN/Code/Data processing/Current in the motor ==
  Data Type Conversion1 : DataTypeConversion
  Divide : Product  Inputs=*/
  Gain1 : Gain  Gain=2/10
  Product1 : Product
  Read Calibration : CoderSF_BSW_Libs/Calibration & Measurement/Read Calibration  variable_name=I_device  variable_value=0  variable_type=single  variable_min=[]  variable_max=[]  unitStr=""  descStr=""
      settings: AttributesFormatString=value:%<variable_value> type:%<variable_type> max:%<variable_max> Min:%<variable_min>
  Read Calibration1 : CoderSF_BSW_Libs/Calibration & Measurement/Read Calibration  variable_name=I_act_filt  variable_value=0  variable_type=int16  variable_min=[]  variable_max=[]  unitStr=""  descStr=""
      settings: AttributesFormatString=value:%<variable_value> type:%<variable_type> max:%<variable_max> Min:%<variable_min>
  Read Calibration4 : CoderSF_BSW_Libs/Calibration & Measurement/Read Calibration  variable_name=I_200  variable_value=0  variable_type=int16  variable_min=[]  variable_max=[]  unitStr=""  descStr=""
      settings: AttributesFormatString=value:%<variable_value> type:%<variable_type> max:%<variable_max> Min:%<variable_min>
  Write Measurement : CoderSF_BSW_Libs/Calibration & Measurement/Write Measurement  variable_name=I_act_filt_A  variable_value=0  variable_type=int16  numD=1  unitStr=A  descStr=""
      settings: AttributesFormatString=type:%<variable_type> Dimensions:%<numD>
  wires:
  Product1/1 -> Data Type Conversion1/1
  Divide/1 -> Product1/2
  Read Calibration4/1 -> Divide/2
  Gain1/1 -> Product1/1
  Read Calibration1/1 -> Divide/1
  Data Type Conversion1/1 -> Write Measurement/1
  Read Calibration/1 -> Gain1/1

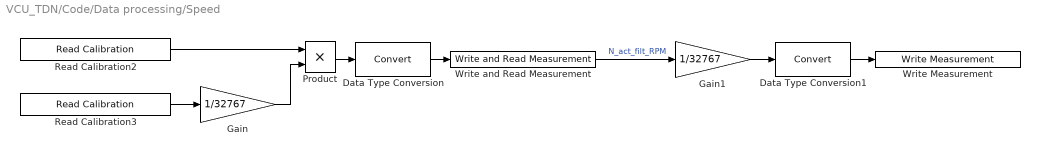
== system VCU_TDN/Code/Data processing/Speed ==
  Data Type Conversion : DataTypeConversion
  Data Type Conversion1 : DataTypeConversion
  Gain : Gain  Gain=1/32767
  Gain1 : Gain  Gain=1/32767
  Product : Product
  Read Calibration2 : CoderSF_BSW_Libs/Calibration & Measurement/Read Calibration  variable_name=SpeedRPMmax  variable_value=0  variable_type=int16  variable_min=[]  variable_max=[]  unitStr=""  descStr=""
      settings: AttributesFormatString=value:%<variable_value> type:%<variable_type> max:%<variable_max> Min:%<variable_min>
  Read Calibration3 : CoderSF_BSW_Libs/Calibration & Measurement/Read Calibration  variable_name=N_act_filt  variable_value=0  variable_type=int16  variable_min=[]  variable_max=[]  unitStr=""  descStr=""
      settings: AttributesFormatString=value:%<variable_value> type:%<variable_type> max:%<variable_max> Min:%<variable_min>
  Write Measurement : CoderSF_BSW_Libs/Calibration & Measurement/Write Measurement  variable_name=Speed  variable_value=0  variable_type=int16  numD=1  unitStr=km/h  descStr=""
      settings: AttributesFormatString=type:%<variable_type> Dimensions:%<numD>
  Write and Read Measurement : CoderSF_BSW_Libs/Calibration & Measurement/Write and Read Measurement  variable_name=N_act_filt_RPM  variable_value=0  variable_type=int16  numD=1  unitStr=RPM  descStr=""
      settings: AttributesFormatString=type:%<variable_type> Dimensions:%<numD>
  wires:
  Read Calibration2/1 -> Product/1
  Read Calibration3/1 -> Gain/1
  Gain/1 -> Product/2
  Product/1 -> Data Type Conversion/1
  Data Type Conversion/1 -> Write and Read Measurement/1
  Write and Read Measurement/1 -> Gain1/1  "N_act_filt_RPM"
  Gain1/1 -> Data Type Conversion1/1
  Data Type Conversion1/1 -> Write Measurement/1

== system VCU_TDN/Code/Initialization/Disabling the inverter ==
  Constant : Constant  Value=hex2dec('51')  OutDataTypeStr=uint8
  Constant1 : Constant  Value=hex2dec('0004')  OutDataTypeStr=uint16
  Pack Signals To CAN Data : CoderSF_BSW_Libs/CAN/Pack Signals To CAN Data  Signal="{{'REG_ID'  'Data1'},[0 8],[8 16],{'uint8'  'uint16'},{'Intel' 'Intel'}}"
  Send CAN Data : CoderSF_BSW_Libs/CAN/Send CAN Data  channel=CAN_A  txlen=3  txid=hex2dec('201')  frametype=Standard(11-bit ID)  showerror=off
  wires:
  Constant/1 -> Pack Signals To CAN Data/1
  Pack Signals To CAN Data/1 -> Send CAN Data/1
  Constant1/1 -> Pack Signals To CAN Data/2

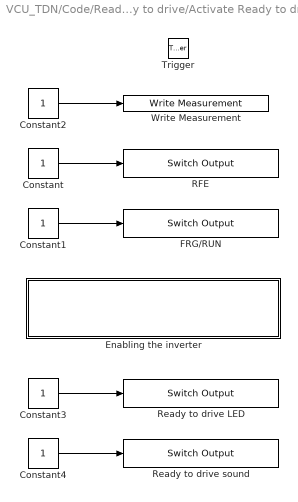
== system VCU_TDN/Code/Ready to drive/Activate Ready to drive ==
  Trigger : TriggerPort  VariantControl=Variant
  Constant{,1..4} (5 alike) : Constant  OutDataTypeStr=boolean
  Enabling the inverter : Subsystem
  FRG/RUN : CoderSF_BSW_Libs/Digital I//O/Switch Output  channel=LSO07
  RFE : CoderSF_BSW_Libs/Digital I//O/Switch Output  channel=LSO06
  Ready to drive LED : CoderSF_BSW_Libs/Digital I//O/Switch Output  channel=LSO08
  Ready to drive sound : CoderSF_BSW_Libs/Digital I//O/Switch Output  channel=LSO10
  Write Measurement : CoderSF_BSW_Libs/Calibration & Measurement/Write Measurement  variable_name=RDY_DRV  variable_value=0  variable_type=boolean  numD=1  unitStr=""  descStr=""
      settings: AttributesFormatString=type:%<variable_type> Dimensions:%<numD>
  wires:
  Constant1/1 -> FRG/RUN/1
  Constant/1 -> RFE/1
  Constant2/1 -> Write Measurement/1
  Constant3/1 -> Ready to drive LED/1
  Constant4/1 -> Ready to drive sound/1

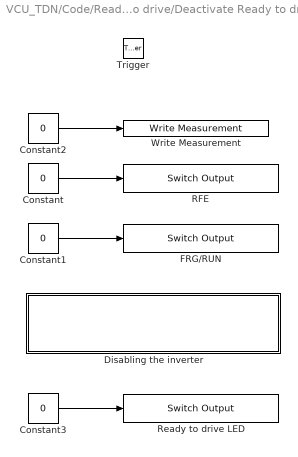
== system VCU_TDN/Code/Ready to drive/Deactivate Ready to drive ==
  Trigger : TriggerPort  VariantControl=Variant
  Constant{,1..3} (4 alike) : Constant  Value=0  OutDataTypeStr=boolean
  Disabling the inverter : Subsystem
  FRG/RUN : CoderSF_BSW_Libs/Digital I//O/Switch Output  channel=LSO07
  RFE : CoderSF_BSW_Libs/Digital I//O/Switch Output  channel=LSO06
  Ready to drive LED : CoderSF_BSW_Libs/Digital I//O/Switch Output  channel=LSO08
  Write Measurement : CoderSF_BSW_Libs/Calibration & Measurement/Write Measurement  variable_name=RDY_DRV  variable_value=0  variable_type=boolean  numD=1  unitStr=""  descStr=""
      settings: AttributesFormatString=type:%<variable_type> Dimensions:%<numD>
  wires:
  Constant1/1 -> FRG/RUN/1
  Constant/1 -> RFE/1
  Constant2/1 -> Write Measurement/1
  Constant3/1 -> Ready to drive LED/1

== system VCU_TDN/Code/Ready to drive/Stop RTD sound ==
  Trigger : TriggerPort  VariantControl=Variant
  Constant4 : Constant  Value=0  OutDataTypeStr=boolean
  Ready to drive sound : CoderSF_BSW_Libs/Digital I//O/Switch Output  channel=LSO10
  wires:
  Constant4/1 -> Ready to drive sound/1

== system VCU_TDN/Code/Receiving data/BMS ==

== system VCU_TDN/Code/Receiving data/Battery temperature sensors ==

== system VCU_TDN/Code/Receiving data/Inverter ==
  Data saving : Subsystem  TreatAsAtomicUnit=on
  Read CAN Message : SF_CanService_Libs/Read CAN Message  typeCAN=Connected  channel=CAN_A  mEn=off  msgInfo=can  msgIterm=INV_VCU  msgItermStore=INV_VCU  valid=on  stale=off  motoBit=off  setSignalName=off  flgCustomMonitorVariableRules=on  defineSignalName=off  prefixSignal='rx'  flgValTest=off  flgNoFixed=on  tSample=Task_L1ms  modeCode=Parameterless
  wires:
  Read CAN Message/1 -> Data saving/Trigger
  Read CAN Message/3 -> Data saving/2(Data)
  Read CAN Message/2 -> Data saving/1(RegID)

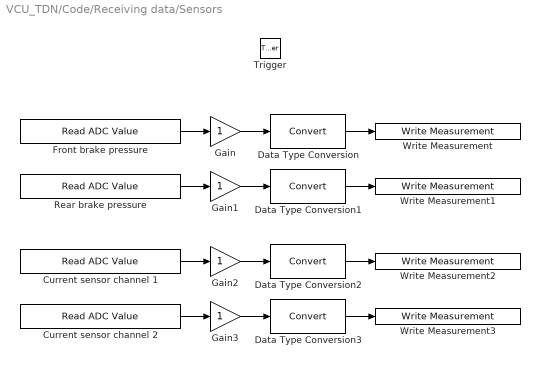
== system VCU_TDN/Code/Receiving data/Sensors ==
  Trigger : TriggerPort  TriggerType=function-call  VariantControl=Variant  PortDimensions=1
  Current sensor channel 1 : CoderSF_BSW_Libs/ADC/Read ADC Value  channel=15
  Current sensor channel 2 : CoderSF_BSW_Libs/ADC/Read ADC Value  channel=17
  Data Type Conversion{,1..3} (4 alike) : DataTypeConversion
  Front brake pressure : CoderSF_BSW_Libs/ADC/Read ADC Value  channel=8
  Gain{,1..3} (4 alike) : Gain
  Rear brake pressure : CoderSF_BSW_Libs/ADC/Read ADC Value  channel=12
  Write Measurement : CoderSF_BSW_Libs/Calibration & Measurement/Write Measurement  variable_name=FR_BRK_PRESSURE  variable_value=0  variable_type=single  numD=1  unitStr=bar  descStr=""
      settings: AttributesFormatString=type:%<variable_type> Dimensions:%<numD>
  Write Measurement1 : CoderSF_BSW_Libs/Calibration & Measurement/Write Measurement  variable_name=RR_BRAKE_PRESSURE  variable_value=0  variable_type=single  numD=1  unitStr=bar  descStr=""
      settings: AttributesFormatString=type:%<variable_type> Dimensions:%<numD>
  Write Measurement2 : CoderSF_BSW_Libs/Calibration & Measurement/Write Measurement  variable_name=CURRENT_CH_1  variable_value=0  variable_type=int16  numD=1  unitStr=A  descStr=""
      settings: AttributesFormatString=type:%<variable_type> Dimensions:%<numD>
  Write Measurement3 : CoderSF_BSW_Libs/Calibration & Measurement/Write Measurement  variable_name=CURRENT_CH_2  variable_value=0  variable_type=int16  numD=1  unitStr=A  descStr=""
      settings: AttributesFormatString=type:%<variable_type> Dimensions:%<numD>
  wires:
  Current sensor channel 2/1 -> Gain3/1
  Current sensor channel 1/1 -> Gain2/1
  Rear brake pressure/1 -> Gain1/1
  Front brake pressure/1 -> Gain/1
  Data Type Conversion/1 -> Write Measurement/1
  Data Type Conversion3/1 -> Write Measurement3/1
  Gain2/1 -> Data Type Conversion2/1
  Data Type Conversion2/1 -> Write Measurement2/1
  Gain1/1 -> Data Type Conversion1/1
  Data Type Conversion1/1 -> Write Measurement1/1
  Gain/1 -> Data Type Conversion/1
  Gain3/1 -> Data Type Conversion3/1

== system VCU_TDN/Code/Ready to drive/Activate Ready to drive/Enabling the inverter ==
  Constant : Constant  Value=hex2dec('51')  OutDataTypeStr=uint8
  Constant1 : Constant  Value=hex2dec('0000')  OutDataTypeStr=uint16
  Pack Signals To CAN Data : CoderSF_BSW_Libs/CAN/Pack Signals To CAN Data  Signal="{{'REG_ID'  'Data1'},[0 8],[8 16],{'uint8'  'uint16'},{'Intel' 'Intel'}}"
  Send CAN Data : CoderSF_BSW_Libs/CAN/Send CAN Data  channel=CAN_A  txlen=3  txid=hex2dec('201')  frametype=Standard(11-bit ID)  showerror=off
  wires:
  Constant/1 -> Pack Signals To CAN Data/1
  Pack Signals To CAN Data/1 -> Send CAN Data/1
  Constant1/1 -> Pack Signals To CAN Data/2

== system VCU_TDN/Code/Ready to drive/Deactivate Ready to drive/Disabling the inverter ==
  Constant : Constant  Value=hex2dec('51')  OutDataTypeStr=uint8
  Constant1 : Constant  Value=hex2dec('0004')  OutDataTypeStr=uint16
  Pack Signals To CAN Data : CoderSF_BSW_Libs/CAN/Pack Signals To CAN Data  Signal="{{'REG_ID'  'Data1'},[0 8],[8 16],{'uint8'  'uint16'},{'Intel' 'Intel'}}"
  Send CAN Data : CoderSF_BSW_Libs/CAN/Send CAN Data  channel=CAN_A  txlen=3  txid=hex2dec('201')  frametype=Standard(11-bit ID)  showerror=off
  wires:
  Constant/1 -> Pack Signals To CAN Data/1
  Pack Signals To CAN Data/1 -> Send CAN Data/1
  Constant1/1 -> Pack Signals To CAN Data/2

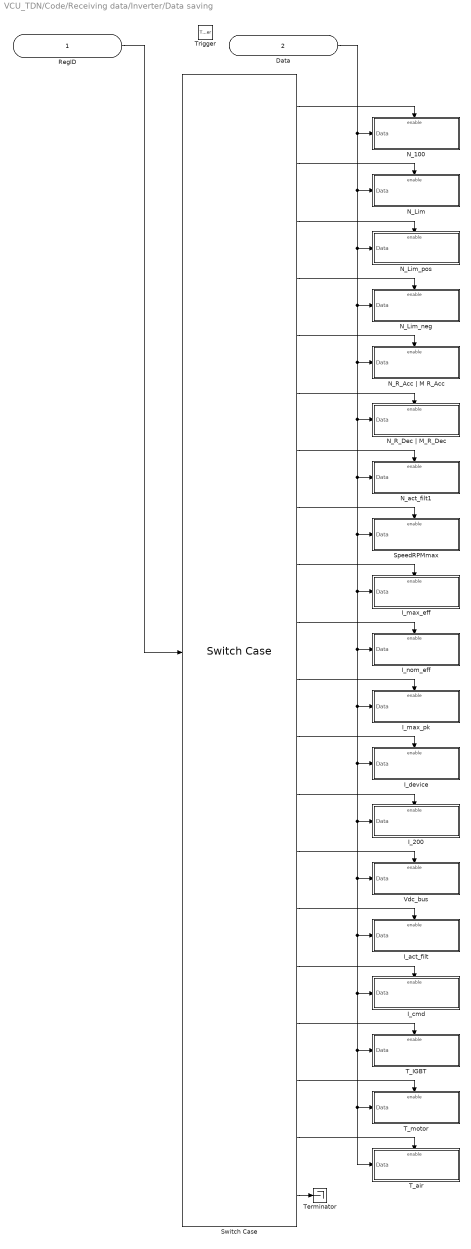
== system VCU_TDN/Code/Receiving data/Inverter/Data saving ==
  RegID : Inport
  Data : Inport  Port=2
  Trigger : TriggerPort  VariantControl=Variant
  I_200 : Subsystem  TreatAsAtomicUnit=on
  I_act_filt : Subsystem  TreatAsAtomicUnit=on
  I_cmd : Subsystem  TreatAsAtomicUnit=on
  I_device : Subsystem  TreatAsAtomicUnit=on
  I_max_eff : Subsystem  TreatAsAtomicUnit=on
  I_max_pk : Subsystem  TreatAsAtomicUnit=on
  I_nom_eff : Subsystem  TreatAsAtomicUnit=on
  N_100 : Subsystem  TreatAsAtomicUnit=on
  N_Lim : Subsystem  TreatAsAtomicUnit=on
  N_Lim_neg : Subsystem  TreatAsAtomicUnit=on
  N_Lim_pos : Subsystem  TreatAsAtomicUnit=on
  N_R_Acc | M R_Acc : Subsystem  TreatAsAtomicUnit=on
  N_R_Dec | M_R_Dec : Subsystem  TreatAsAtomicUnit=on
  N_act_filt1 : Subsystem  TreatAsAtomicUnit=on
  SpeedRPMmax : Subsystem  TreatAsAtomicUnit=on
  Switch Case : SwitchCase  CaseConditions={0xc8,0x34,0x3f,0x3e,0x35,0xed,0xce,0xa8,0x4d,0x4e,0xc4,0xc6,0xd9,0xeb,0x5f,0x26,0x4a,0x49,0x4b}
  T_IGBT : Subsystem  TreatAsAtomicUnit=on
  T_air : Subsystem  TreatAsAtomicUnit=on
  T_motor : Subsystem  TreatAsAtomicUnit=on
  Terminator : Terminator
  Vdc_bus : Subsystem  TreatAsAtomicUnit=on
  wires:
  RegID/1 -> Switch Case/1
  Data/1 -> N_R_Dec | M_R_Dec/1(Data), N_act_filt1/1(Data), I_device/1(Data), I_200/1(Data), Vdc_bus/1(Data), T_air/1(Data), T_motor/1(Data), T_IGBT/1(Data), I_cmd/1(Data), I_act_filt/1(Data), I_max_pk/1(Data), I_nom_eff/1(Data), I_max_eff/1(Data), SpeedRPMmax/1(Data), N_R_Acc | M R_Acc/1(Data), N_Lim_neg/1(Data), N_Lim_pos/1(Data), N_Lim/1(Data), N_100/1(Data)
  Switch Case/1 -> N_100/Enable
  Switch Case/2 -> N_Lim/Enable
  Switch Case/3 -> N_Lim_pos/Enable
  Switch Case/4 -> N_Lim_neg/Enable
  Switch Case/5 -> N_R_Acc | M R_Acc/Enable
  Switch Case/6 -> N_R_Dec | M_R_Dec/Enable
  Switch Case/7 -> N_act_filt1/Enable
  Switch Case/8 -> SpeedRPMmax/Enable
  Switch Case/9 -> I_max_eff/Enable
  Switch Case/10 -> I_nom_eff/Enable
  Switch Case/11 -> I_max_pk/Enable
  Switch Case/12 -> I_device/Enable
  Switch Case/13 -> I_200/Enable
  Switch Case/14 -> Vdc_bus/Enable
  Switch Case/15 -> I_act_filt/Enable
  Switch Case/16 -> I_cmd/Enable
  Switch Case/17 -> T_IGBT/Enable
  Switch Case/18 -> T_motor/Enable
  Switch Case/19 -> T_air/Enable
  Switch Case/20 -> Terminator/1

== system VCU_TDN/Code/Receiving data/Inverter/Data saving/I_200 ==
  Data : Inport
  Enable : EnablePort
  Data Type Conversion : DataTypeConversion
  Write Measurement : CoderSF_BSW_Libs/Calibration & Measurement/Write Measurement  variable_name=I_200  variable_value=0  variable_type=int16  numD=1  unitStr=""  descStr=""
      settings: AttributesFormatString=type:%<variable_type> Dimensions:%<numD>
  wires:
  Data Type Conversion/1 -> Write Measurement/1
  Data/1 -> Data Type Conversion/1
